simulink model "SimulationFile"  (R2024a)
settings: Solver=VariableStepAuto  StartTime=0.0  StopTime=10  MaxStep=100e-6  RelTol=1e-3
values from neighbouring files (symbols this model uses):
  D = D_values(i)    [main.m]    (also in poles_damping_inductance.m; poles_inductance.m; poles_inductance_damping.m; poles_renewable_resistance.m = Dth)
  H = 1    [main.m]    (also in poles_damping_inductance.m; poles_inductance.m; poles_inductance_damping.m; poles_renewable_resistance.m)
  L2 = L^2    (= 0.01)    [main.m]    (also in poles_damping_inductance.m; poles_inductance.m = L^2; poles_inductance_damping.m = L^2; poles_renewable_resistance.m)
  omega_s = 2*pi*fs    (= 314.159265359)    [main.m]    (also in plot_poles_renewables_resistance.m; poles_damping_inductance.m; poles_inductance.m; poles_inductance_damping.m)
  Pref = 3*V^2*R/(R^2 + (omega_s*L)^2)    [main.m]    (also in poles_damping_inductance.m; poles_inductance.m; poles_inductance_damping.m; poles_renewable_resistance.m)
  R = R_values(k)    [main.m]    (also in poles_damping_inductance.m; poles_inductance.m = 100; poles_inductance_damping.m = 100; poles_renewable_resistance.m = Values(k))
  R2 = R^2    [main.m]    (also in poles_damping_inductance.m; poles_inductance.m = 10000; poles_inductance_damping.m = 10000; poles_renewable_resistance.m)
  V2 = V^2    (= 10000)    [main.m]    (also in poles_damping_inductance.m; poles_inductance.m; poles_inductance_damping.m; poles_renewable_resistance.m)
settings Model: Creator=yoashl  LastModifiedBy=elino
settings SolverCC: AlgebraicLoopSolver=TrustRegion
settings DebuggingCC: UnconnectedInputMsg=warning  UnconnectedOutputMsg=warning  UnconnectedLineMsg=warning
settings ModelReferenceCC: EnableRefExpFcnMdlSchedulingChecks=on
settings RTWCC: GPUComputeCapability=3.5

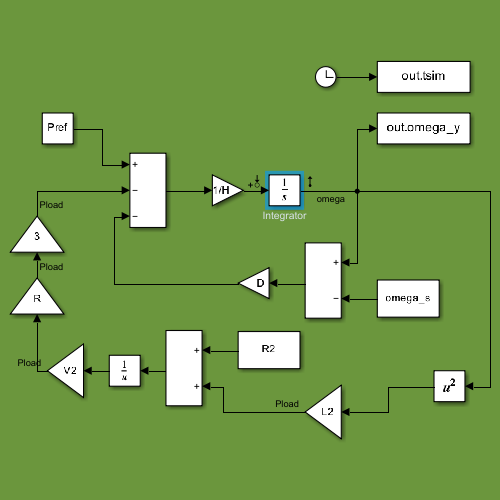
[thumbnail: Simulink's stored preview of the top-level diagram]
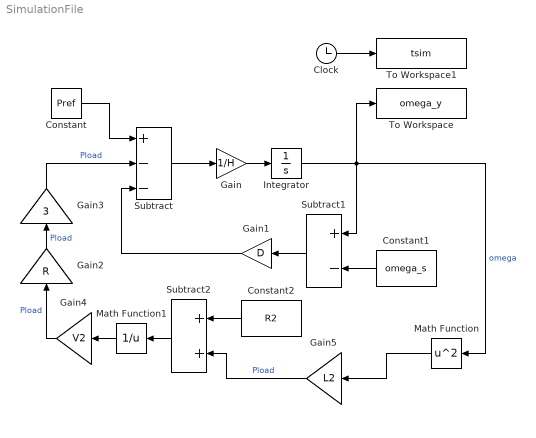
== system SimulationFile ==
  Clock : Clock
  Constant : Constant  Value=Pref
  Constant1 : Constant  Value=omega_s
  Constant2 : Constant  Value=R2
  Gain : Gain  Gain=1/H
  Gain1 : Gain  Gain=D
  Gain2 : Gain  Gain=R
  Gain3 : Gain  Gain=3
  Gain4 : Gain  Gain=V2
  Gain5 : Gain  Gain=L2
  Integrator : Integrator  InitialCondition=omega_s*0.5
  Math Function : Math  Operator=square
  Math Function1 : Math  Operator=reciprocal
  Subtract : Sum  Inputs=+--
  Subtract1 : Sum  Inputs=+-
  Subtract2 : Sum
  To Workspace : ToWorkspace  VariableName=omega_y  SampleTime=-1
  To Workspace1 : ToWorkspace  VariableName=tsim  SampleTime=-1
  wires:
  Subtract/1 -> Gain/1
  Constant/1 -> Subtract/1
  Integrator/1 -> To Workspace/1, Math Function/1, Subtract1/1  "omega"
  Subtract1/1 -> Gain1/1
  Gain1/1 -> Subtract/3
  Constant1/1 -> Subtract1/2
  Gain2/1 -> Gain3/1  "Pload"
  Gain3/1 -> Subtract/2  "Pload"
  Gain4/1 -> Gain2/1  "Pload"
  Constant2/1 -> Subtract2/1
  Math Function/1 -> Gain5/1
  Gain5/1 -> Subtract2/2  "Pload"
  Math Function1/1 -> Gain4/1
  Subtract2/1 -> Math Function1/1
  Clock/1 -> To Workspace1/1
  Gain/1 -> Integrator/1
